simulink model "switched_simstate_tf"  (R2020a)
settings: Solver=FixedStepAuto  StartTime=22  StopTime=42  FixedStep=dt  RelTol=1e-3
values from neighbouring files (symbols this model uses):
  dt = 0.001    [param_init.m]    (also in sim_switched.m = options.dt)
libraries: simulink x1
settings Model: Creator=kekatos  LastModifiedBy=kekatos
settings DataIOCC: FinalStateName=SimState  InitialState=SimState_previous  LoadInitialState=on  SaveFinalState=on  SaveOperatingPoint=on  DSMLogging=off  ReturnWorkspaceOutputs=off

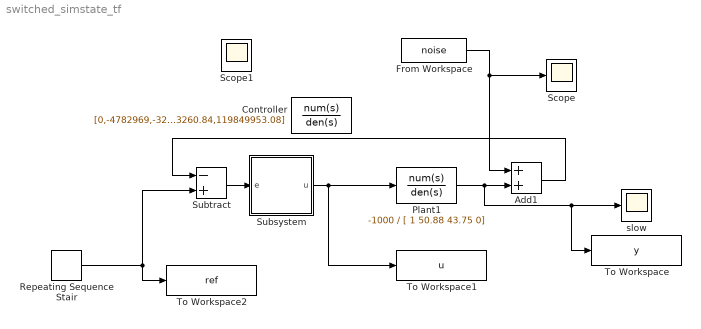
== system switched_simstate_tf ==
  Add1 : Sum
  Controller : TransferFcn  Numerator=[0,-4782969,-321787153.4913,-316286050.3938]  Denominator=[1,974.2,473260.84,119849953.08]
  From Workspace : FromWorkspace  VariableName=noise
  Plant1 : TransferFcn  Numerator=-1000  Denominator=[ 1 50.88 43.75 0]
  Repeating Sequence Stair : simulink/Sources/Repeating Sequence Stair  OutValues=[1 1 1 1 1 0 0 0 0 0 2 2].'  tsamp=2  OutMin=[]  OutMax=[]  OutDataTypeStr=double  OutputDataTypeScalingMode=double  OutDataType=fixdt(0,8)  ConRadixGroup=Best Precision: Vector-wise  OutScaling=2^-12
  Scope : Scope
  Subsystem : Subsystem
  Subtract : Sum  Inputs=-+
  To Workspace : ToWorkspace  VariableName=y  SaveFormat=Structure With Time  SampleTime=dt
  To Workspace1 : ToWorkspace  VariableName=u  SaveFormat=Structure With Time  SampleTime=dt
  To Workspace2 : ToWorkspace  VariableName=ref  SaveFormat=Structure With Time  SampleTime=dt
  slow : Scope
  Scope1 : Scope
  wires:
  Plant1/1 -> To Workspace/1, slow/1, Add1/2
  Repeating Sequence Stair/1 -> To Workspace2/1, Subtract/2
  Add1/1 -> Subtract/1
  From Workspace/1 -> Scope/1, Add1/1
  Subtract/1 -> Subsystem/1(e)
  Subsystem/1(u) -> Plant1/1, To Workspace1/1

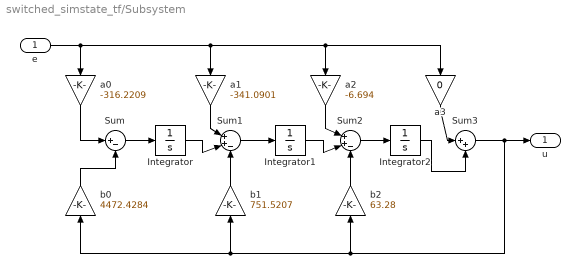
== system switched_simstate_tf/Subsystem ==
  e : Inport
  Integrator : Integrator
  Integrator1 : Integrator
  Integrator2 : Integrator
  Sum : Sum  Inputs=|+-
  Sum1 : Sum  Inputs=|++-
  Sum2 : Sum  Inputs=|++-
  Sum3 : Sum  Inputs=|++
  a0 : Gain  Gain=-316.2209
  a1 : Gain  Gain=-341.0901
  a2 : Gain  Gain=-6.694
  a3 : Gain  Gain=0
  b0 : Gain  Gain=4472.4284
  b1 : Gain  Gain=751.5207
  b2 : Gain  Gain=63.28
  u : Outport
  wires:
  Sum/1 -> Integrator/1
  a0/1 -> Sum/1
  b0/1 -> Sum/2
  Integrator/1 -> Sum1/2
  a1/1 -> Sum1/1
  Sum3/1 -> b2/1, b1/1, b0/1, u/1
  Sum1/1 -> Integrator1/1
  a2/1 -> Sum2/1
  Integrator1/1 -> Sum2/2
  b1/1 -> Sum1/3
  b2/1 -> Sum2/3
  e/1 -> a3/1, a2/1, a1/1, a0/1
  Integrator2/1 -> Sum3/2
  a3/1 -> Sum3/1
  Sum2/1 -> Integrator2/1
